simulink model "BitClear1"  (R2017b)
settings: Solver=FixedStepDiscrete  StartTime=0.0  StopTime=19.8  FixedStep=0.200000  RelTol=1e-3
model workspace (MAT data in the model file):
  already_pp = 0
  input_dataset = Simulink.SimulationData.Dataset
  input_dataset.any.Name = ''
  input_dataset.any.Version = 3
  input_dataset.any.Storage = Simulink.SimulationData.Storage.RamDatasetStorage
  input_dataset.any.Storage.any.Version = 2
  input_dataset.any.Storage.any.Elements{1} = Simulink.SimulationData.Signal
  input_dataset.any.Storage.any.Elements{1}.Version = 1
  input_dataset.any.Storage.any.Elements{1}.Values = timeseries
  input_dataset.any.Storage.any.Elements{1}.Values.Name = 'unnamed'
  input_dataset.any.Storage.any.Elements{1}.Values.DataInfo = tsdata.datametadata
  input_dataset.any.Storage.any.Elements{1}.Values.DataInfo.Interpolation = tsdata.interpolation
  input_dataset.any.Storage.any.Elements{1}.Values.DataInfo.Interpolation.Fhandle : function handle (value not decoded)
  input_dataset.any.Storage.any.Elements{1}.Values.DataInfo.Interpolation.Name = 'linear'
  input_dataset.any.Storage.any.Elements{1}.Values.TimeInfo = tsdata.timemetadata
  input_dataset.any.Storage.any.Elements{1}.Values.TimeInfo.Length = 100
  input_dataset.any.Storage.any.Elements{1}.Values.TimeInfo.DuplicateTimes = 0
  input_dataset.any.Storage.any.Elements{1}.Values.TimeInfo.Time_ = [0; 0.2; 0.4; 0.6; 0.8; 1; 1.2; 1.4; 1.6; 1.8; 2; 2.2; 2.4; 2.6; 2.8; 3; 3.2; 3.4; 3.6; 3.8; 4; 4.2; 4.4; 4.6; 4.8; 5; 5.2; 5.4; 5.6; 5.8; 6; 6.2; 6.4; 6.6; 6.8; 7; 7.2; 7.4; 7.6; 7.8; 8; 8.2; 8.4; 8.6; 8.8; 9; 9.2; 9.4; 9.6; 9.8; 10; 10.2; 10.4; 10.6; 10.8; 11; 11.2; 11.4; 11.6; 11.8; 12; 12.2; 12.4; 12.6; 12.8; 13; 13.2; 13.4; 13.6; 13.8; 14; 14.2; 14.4; 14.6; 14.8; 15; 15.2; 15.4; 15.6; 15.8; 16; 16.2; 16.4; 16.6; 16.8; 17; 17.2; 17.4; 17.6; 17.8; 18; 18.2; 18.4; 18.6; 18.8; 19; 19.2; 19.4; 19.6; 19.8]
  input_dataset.any.Storage.any.Elements{1}.Values.TimeInfo.Initialized = 1
  input_dataset.any.Storage.any.Elements{1}.Values.QualityInfo = tsdata.qualmetadata
  input_dataset.any.Storage.any.Elements{1}.Values.Data_ = [-160; -83; 80; 292; -176; 155; 232; -17; -205; 187; -14; -231; 226; 81; -242; 245; -279; -277; 294; 112; -74; 3; 158; -271; 136; 121; -25; 49; -97; -198; -61; 252; -165; -84; -105; -250; 8; 200; 243; 134; -70; -121; 115; 229; 255; -252; -10; -223; -149; 231; -183; -228; 26; -111; -71; 175; 204; 108; -50; 86; -172; 70; 105; 61; -92; -81; -197; 178; -4; -87; 165; -158; 207; 190; 208; -78; -70; 217; -22; 42; 117; 277; 28; 82; 43; 257; 219; -198; -193; -154; 151; -181; 290; 126; -195; 215; 246; 277; 42; 38]
  input_dataset.any.Storage.any.Elements{1}.Name = 'u'
settings Model: Creator=hbourbou  LastModifiedBy=hbourbou
settings DataIOCC: ExternalInput=input_dataset  LoadExternalInput=on  SaveState=on
settings DebuggingCC: AlgebraicLoopMsg=error  ArtificialAlgebraicLoopMsg=error
settings GRTTargetCC: ExtMode=on

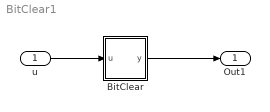
== system BitClear1 ==
  u : Inport  OutDataTypeStr=int32
  BitClear : Subsystem  AncestorBlock=simulink/Logic and Bit Operations/Bit Clear  TreatAsAtomicUnit=on  mask(Bit Clear){iBit=2}
      mask prompts: iBit "Simulink:masks:IndexOfBit0IsLeastSignificant_MP"
      mask help: Simulink:masks:BitClear_MD
      mask init:
      | if length(iBit) == 1
      |   dispStr = sprintf('Clear\nbit %d',double(iBit));
      | else
      |   dispStr=sprintf('Vector\nBit Clear');
      | end
      mask Display: disp(dispStr)
  Out1 : Outport
  wires:
  u/1 -> BitClear/1(u)
  BitClear/1(y) -> Out1/1

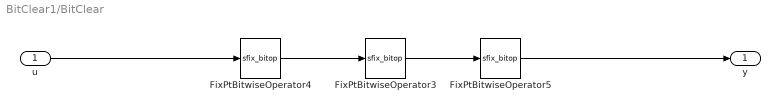
== system BitClear1/BitClear ==
  u : Inport
  FixPtBitwiseOperator3 : S-Function  AncestorBlock=|  FunctionName=sfix_bitop  Parameters=UseBitMask,NumInputPorts,BitMask,BitMaskRealWorld,logicop  SFunctionDeploymentMode=off  EnableBusSupport=off  mask(Bitwise Operator){logicop=OR, UseBitMask=on, NumInputPorts=1, BitMask=2.^double(iBit), BitMaskRealWorld=Stored Integer}
      | simulink/Logic and Bit
      | Operations/Bitwise
      | Operator
      mask prompts: logicop "Simulink:masks:Operator_MP"; UseBitMask "Simulink:masks:UseBitMask_MP"; NumInputPorts "Simulink:masks:NumberOfInputPorts_MP"; BitMask "Simulink:masks:BitMask_MP"; BitMaskRealWorld "Simulink:masks:TreatMaskAs_MP"
      mask help: Simulink:masks:BitwiseOperator_MD
      mask init:
      | str = '';
      | if UseBitMask
      |   [m,n] = size(BitMask);
      |   if ischar(BitMask)
      |     len = m;
      |     n = 1;
      |   else
      |     len = m * n;
      |   end
      |   internalBitMask = zeros(m,n);
      |   if isnumeric(BitMask)
      |     if ~isreal(BitMask)
      |       error(DAStudio.message('Simulink:blocks:BitMaskNotComplex'));
      |     end
      |     for i=1:len,
      |       internalBitMask(i) = BitMask(i);
      |     end
      |   elseif ischar(BitMask)
      |     for i=1:m,
      |       internalBitMask(i) = hex2dec(BitMask(i,:));
      |     end
      |   elseif iscell(BitMask)
      |     for i=1:len,
      |       if isnumeric( BitMask{i} )
      |         internalBitMask(i) = BitMask{i};
      |       elseif ischar( BitMask{i} )
      |         internalBitMask(i) = hex2dec(BitMask{i});
      |       else
      |         errordlg(['Data type is not supported at cell item ', num2str(i) ]);
      |       end
      |     end
      |   end
      |   BitMask = internalBitMask;
      |   for i=1:len
      |     if BitMask(i) > (2^52)-1
      |       error(DAStudio.message('Simulink:blocks:BitMaskWordLengthTooLarge')); 
      |     end
      |   end 
      |   if len == 1
      |      if BitMaskRealWorld == 1 || BitMask(1) < 0
      |        str=num2str(BitMask(1));
      |      else
      |        str=['0x',dec2hex(floor(BitMask(1)))];
      |      end
      |   else
      |      str='Masks';
      |   end
      | else
      |   BitMask = 0;
      |   str='';
      | end
      mask TypeOptions logicop: Simulink:masks:AND | Simulink:masks:OR | Simulink:masks:NAND | Simulink:masks:NOR | Simulink:masks:XOR | Simulink:masks:NOT
      mask Callback logicop: fixptdialog(gcbh)
      mask Callback UseBitMask: fixptdialog(gcbh)
      mask TypeOptions BitMaskRealWorld: Simulink:masks:RealWorldValue | Simulink:masks:StoredInteger
      mask Display: fprintf(['Bitwise\n',logicop,'\n',str])
  FixPtBitwiseOperator4 : S-Function  AncestorBlock=|  FunctionName=sfix_bitop  Parameters=UseBitMask,NumInputPorts,BitMask,BitMaskRealWorld,logicop  SFunctionDeploymentMode=off  EnableBusSupport=off  mask(Bitwise Operator){logicop=NOT, UseBitMask=off, NumInputPorts=1, BitMask=2^iBit, BitMaskRealWorld=Stored Integer}
      | simulink/Logic and Bit
      | Operations/Bitwise
      | Operator
      mask prompts: logicop "Simulink:masks:Operator_MP"; UseBitMask "Simulink:masks:UseBitMask_MP"; NumInputPorts "Simulink:masks:NumberOfInputPorts_MP"; BitMask "Simulink:masks:BitMask_MP"; BitMaskRealWorld "Simulink:masks:TreatMaskAs_MP"
      mask help: Simulink:masks:BitwiseOperator_MD
      mask init: same as BitClear1/BitClear/FixPtBitwiseOperator3
      mask TypeOptions logicop: Simulink:masks:AND | Simulink:masks:OR | Simulink:masks:NAND | Simulink:masks:NOR | Simulink:masks:XOR | Simulink:masks:NOT
      mask Callback logicop: fixptdialog(gcbh)
      mask Callback UseBitMask: fixptdialog(gcbh)
      mask TypeOptions BitMaskRealWorld: Simulink:masks:RealWorldValue | Simulink:masks:StoredInteger
      mask Display: fprintf(['Bitwise\n',logicop,'\n',str])
  FixPtBitwiseOperator5 : S-Function  AncestorBlock=|  FunctionName=sfix_bitop  Parameters=UseBitMask,NumInputPorts,BitMask,BitMaskRealWorld,logicop  SFunctionDeploymentMode=off  EnableBusSupport=off  mask(Bitwise Operator){logicop=NOT, UseBitMask=off, NumInputPorts=1, BitMask=2^iBit, BitMaskRealWorld=Stored Integer}
      | simulink/Logic and Bit
      | Operations/Bitwise
      | Operator
      mask prompts: logicop "Simulink:masks:Operator_MP"; UseBitMask "Simulink:masks:UseBitMask_MP"; NumInputPorts "Simulink:masks:NumberOfInputPorts_MP"; BitMask "Simulink:masks:BitMask_MP"; BitMaskRealWorld "Simulink:masks:TreatMaskAs_MP"
      mask help: Simulink:masks:BitwiseOperator_MD
      mask init: same as BitClear1/BitClear/FixPtBitwiseOperator3
      mask TypeOptions logicop: Simulink:masks:AND | Simulink:masks:OR | Simulink:masks:NAND | Simulink:masks:NOR | Simulink:masks:XOR | Simulink:masks:NOT
      mask Callback logicop: fixptdialog(gcbh)
      mask Callback UseBitMask: fixptdialog(gcbh)
      mask TypeOptions BitMaskRealWorld: Simulink:masks:RealWorldValue | Simulink:masks:StoredInteger
      mask Display: fprintf(['Bitwise\n',logicop,'\n',str])
  y : Outport
  wires:
  FixPtBitwiseOperator5/1 -> y/1
  u/1 -> FixPtBitwiseOperator4/1
  FixPtBitwiseOperator4/1 -> FixPtBitwiseOperator3/1
  FixPtBitwiseOperator3/1 -> FixPtBitwiseOperator5/1
